simulink model "matlab model"  (R2023a)
settings: Solver=ode4  StartTime=0.0  StopTime=0.15  FixedStep=1e-6  RelTol=1e-3  EnableMultiTasking=on
libraries: neural x15, spsMosfetLib x15, simulink x10, spsMeanLib x6, spsSeriesRLCBranchLib x4, spsVoltageMeasurementLib x3, spsDCVoltageSourceLib x2, spsThreePhaseVIMeasurementLib x1, sps_lib x1
(part 1 of 2)
settings Model: Creator=VENUS  LastModifiedBy=air
settings SolverCC: AlgebraicLoopSolver=TrustRegion
settings DataIOCC: LimitDataPoints=on  SaveFormat=Array  ReturnWorkspaceOutputs=off
settings OptimizationCC: LifeSpan=inf
settings DebuggingCC: SolverPrmCheckMsg=warning  UnconnectedInputMsg=warning  UnconnectedOutputMsg=warning  UnconnectedLineMsg=warning  SFUnexpectedBacktrackingDiag=warning  SFNoUnconditionalDefaultTransitionDiag=warning  SFExecutionAtInitializationDiag=none  ArithmeticOperatorsInVariantConditions=warning
settings HardwareCC: ProdBitPerPointer=32  ProdBitPerSizeT=32  ProdBitPerPtrDiffT=32  ProdLargestAtomicFloat=None  ProdIntDivRoundTo=Undefined  ProdEndianess=Unspecified  ProdWordSize=32  ProdHWDeviceType=32-bit Generic
settings ModelReferenceCC: EnableRefExpFcnMdlSchedulingChecks=on  PropagateSignalLabelsOutOfModel=off
settings SFSimCC: SimUseLocalCustomCode=off  CustomCodeUndefinedFunction=UseInterfaceOnly
settings RTWCC: RTWUseLocalCustomCode=off
settings CodeAppCC: StateflowObjectComments=on
settings GRTTargetCC: TargetLangStandard=C89/C90 (ANSI)
settings ConfigComp: CovMetricSettings=dw  CovSaveCumulativeToWorkspaceVar=on  CovSaveSingleToWorkspaceVar=on  CovExternalEMLEnable=off  CovSFcnEnable=off
settings SimscapeCC: SimscapeNormalizeSystem=off

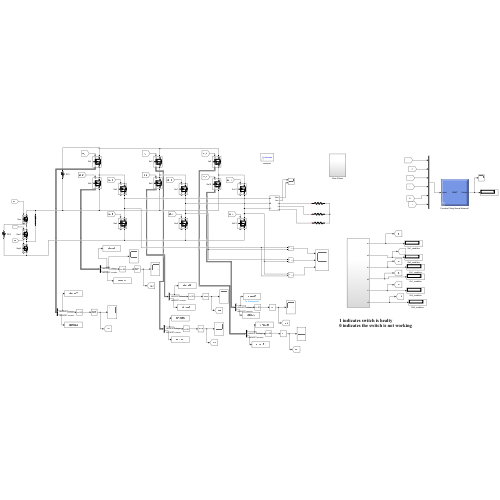
[thumbnail: Simulink's stored preview of the top-level diagram]
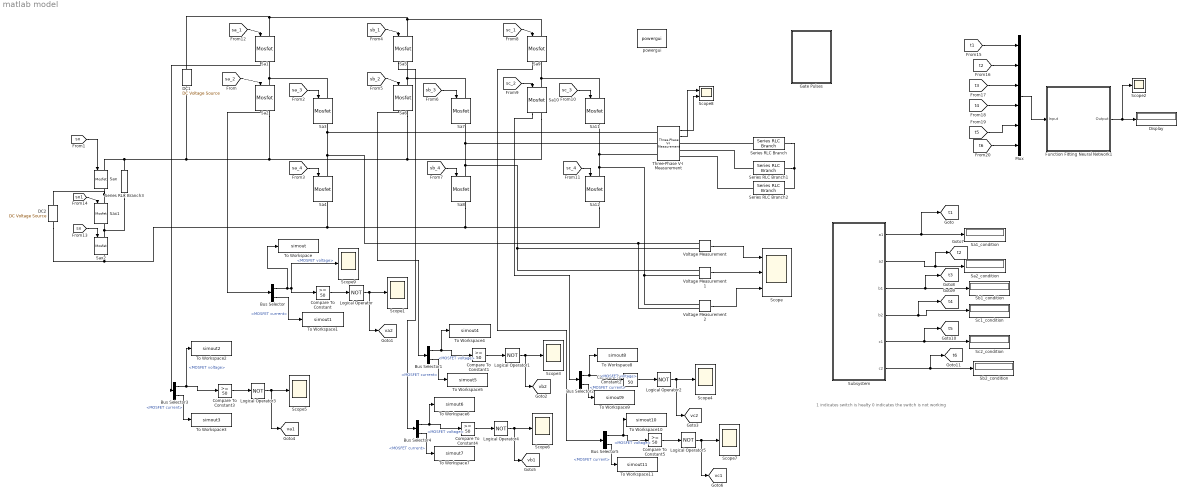
== system matlab model ==
  note: 1 indicates switch is healty
      | 0 indicates the switch is not working
  Bus Selector{,1..5} (6 alike) : BusSelector  OutputSignals=MOSFET voltage,MOSFET current
  Compare To Constant{,1..5} (6 alike) : simulink/Logic and Bit Operations/Compare To Constant  relop=>=  const=50  OutDataTypeStr=boolean
  DC1 : spsDCVoltageSourceLib/DC Voltage Source  Amplitude=300  Measurements=None
  DC2 : spsDCVoltageSourceLib/DC Voltage Source  Amplitude=300  Measurements=None
  Display : Display
  Function Fitting Neural Network1 : Subsystem
      mask help: Function Fitting Neural Network
      mask Display: e = 0.06;c1 = [120 150 230]/255;c2 = ([120 150 230]+0)/383;c3 = ([120 150 230]+128)/383;patch([0 1 1 0],[0 0 1 1],c1);patch([0 1 1 1-e 1-e 0+e],[0 0 1 1-e 0+e 0+e],c2);patch([0 0 1 1-e 0+e 0+e],[0 1 1 1-e 1-e 0+e],c3);plot([0 1 1 0 0],[0 0 1 1 0]);fprintf('NNET');port_label('input',1,' Input');port_label('output',1,'Output ');
  Gate Pulses : Subsystem
  Logical Operator{,1..5} (6 alike) : Logic  Operator=NOT  AllPortsSameDT=off  OutDataTypeStr=boolean
  Mux : Mux  Inputs=6
  Sa{1..12} (12 alike) : spsMosfetLib/Mosfet  Ron=0.1  Lon=0  Rd=0.01  Vfd=0  IC=0  Rs=1e5  Cs=inf  Measurements=on
  Sa1_condition : Display
  Sa2_condition : Display
  Sax : spsMosfetLib/Mosfet  Ron=0.1  Lon=0  Rd=0.01  Vfd=0  IC=0  Rs=1e5  Cs=inf  Measurements=on
  Sax1 : spsMosfetLib/Mosfet  Ron=0.1  Lon=0  Rd=0.01  Vfd=0  IC=0  Rs=1e5  Cs=inf  Measurements=on
  Sax2 : spsMosfetLib/Mosfet  Ron=0.1  Lon=0  Rd=0.01  Vfd=0  IC=0  Rs=1e5  Cs=inf  Measurements=on
  Sb1_condition : Display
  Sb2_condition : Display
  Sc1_condition : Display
  Sc2_condition : Display
  Scope : Scope  NumInputPorts=3
  Scope{1..7,9} (8 alike) : Scope
  Scope8 : Scope  NumInputPorts=2
  Series RLC Branch : spsSeriesRLCBranchLib/Series RLC Branch  LConnTagsString=__new0  RConnTagsString=__new0  BranchType=R  Resistance=100  Inductance=1e-3  SetiL0=off  InitialCurrent=0  Capacitance=1e-6  Setx0=off  InitialVoltage=0  Measurements=None
  Series RLC Branch1 : spsSeriesRLCBranchLib/Series RLC Branch  LConnTagsString=__new0  RConnTagsString=__new0  BranchType=R  Resistance=100  Inductance=1e-3  SetiL0=off  InitialCurrent=0  Capacitance=1e-6  Setx0=off  InitialVoltage=0  Measurements=None
  Series RLC Branch2 : spsSeriesRLCBranchLib/Series RLC Branch  LConnTagsString=__new0  RConnTagsString=__new0  BranchType=R  Resistance=100  Inductance=1e-3  SetiL0=off  InitialCurrent=0  Capacitance=1e-6  Setx0=off  InitialVoltage=0  Measurements=None
  Series RLC Branch3 : spsSeriesRLCBranchLib/Series RLC Branch  LConnTagsString=__new0  RConnTagsString=__new0  BranchType=RC  Resistance=0.01  Inductance=1e-3  SetiL0=off  InitialCurrent=0  Capacitance=1000e-6  Setx0=off  InitialVoltage=0  Measurements=None
  Subsystem : Subsystem
  Three-Phase V-I Measurement : spsThreePhaseVIMeasurementLib/Three-Phase V-I Measurement  VoltageMeasurement=phase-to-phase  SetLabelV=off  LabelV=Vabc  Vpu=off  VpuLL=off  CurrentMeasurement=yes  SetLabelI=off  LabelI=Iabc  Ipu=off  Pbase=100e6  Vbase=500e3  OutputType=Complex  PhasorSimulation=off  PSBequivalent=0
  To Workspace : ToWorkspace  VariableName=simout  SaveFormat=Timeseries  SampleTime=-1
  To Workspace1 : ToWorkspace  VariableName=simout1  SaveFormat=Timeseries  SampleTime=-1
  To Workspace10 : ToWorkspace  VariableName=simout10  SaveFormat=Timeseries  SampleTime=-1
  To Workspace11 : ToWorkspace  VariableName=simout11  SaveFormat=Timeseries  SampleTime=-1
  To Workspace2 : ToWorkspace  VariableName=simout2  SaveFormat=Timeseries  SampleTime=-1
  To Workspace3 : ToWorkspace  VariableName=simout3  SaveFormat=Timeseries  SampleTime=-1
  To Workspace4 : ToWorkspace  VariableName=simout4  SaveFormat=Timeseries  SampleTime=-1
  To Workspace5 : ToWorkspace  VariableName=simout5  SaveFormat=Timeseries  SampleTime=-1
  To Workspace6 : ToWorkspace  VariableName=simout6  SaveFormat=Timeseries  SampleTime=-1
  To Workspace7 : ToWorkspace  VariableName=simout7  SaveFormat=Timeseries  SampleTime=-1
  To Workspace8 : ToWorkspace  VariableName=simout8  SaveFormat=Timeseries  SampleTime=-1
  To Workspace9 : ToWorkspace  VariableName=simout9  SaveFormat=Timeseries  SampleTime=-1
  Voltage Measurement : spsVoltageMeasurementLib/Voltage Measurement  PhasorSimulation=off  OutputType=Complex  PSBequivalent=0
  Voltage Measurement1 : spsVoltageMeasurementLib/Voltage Measurement  PhasorSimulation=off  OutputType=Complex  PSBequivalent=0
  Voltage Measurement2 : spsVoltageMeasurementLib/Voltage Measurement  PhasorSimulation=off  OutputType=Complex  PSBequivalent=0
  powergui : sps_lib/powergui  Priority=1  SimulationMode=Continuous  SampleTime=50e-6  frequency=60  Iterations=50  frequencyindice=0  Pbase=100e6  ErrMax=1e-4  UnitsV=kV  UnitsW=MW  buscounter=0  FunctionMessages=off  echomessages=off  EnableUseOfTLC=off  CurrentSourceSwitches=on  DisableSnubberDevices=off  DisableRonSwitches=off  DisableVfSwitches=off  DisplayEquations=off  AutomaticDiscreteSolvers=off  SolverType=Tustin  Interpol=off  ExternalGateDelay=off  methode=off  Ts=0  x0status=blocks  SPID=off  SwTol=0  HookPort=off  NonlinearTolerance=1e-4  nMaxIteration=100  ContinueOnMaxIteration=off  RestoreLinks=warning  ResistiveCurrentMeasurement=off  Frange=[0:2:500]  Ylog=off  Xlog=on  ShowGrid=off  save=off  variable=ZData  structure=0  ZoomFFT=off  StartTime=0.0  cycles=1  DisplayStyle=1  fundamental=60  FreqAxis=off  MaxFrequency=1000  frequencyindicesteady=1  RmsSteady=1  display=off
  tag scope: t1=global, t2=global, t3=global, t4=global, t5=global, t6=global, va1=global, va2=global, vb1=global, vb2=global, vc1=global, vc2=global
  wires:
  [sa_3] -> Sa3/1
  [sa_4] -> Sa4/1
  [sb_4] -> Sa8/1
  [sb_3] -> Sa7/1
  [sb_2] -> Sa6/1
  [sb_1] -> Sa5/1
  [sc_1] -> Sa9/1
  [sc_2] -> Sa10/1
  [sc_4] -> Sa12/1
  [sc_3] -> Sa11/1
  Voltage Measurement1/1 -> Scope/2
  Voltage Measurement/1 -> Scope/1
  Voltage Measurement2/1 -> Scope/3
  Sa2/1 -> Bus Selector/1
  Bus Selector/1 -> To Workspace/1, Compare To Constant/1, Scope9/1  "<MOSFET voltage>"
  Compare To Constant/1 -> Logical Operator/1
  Logical Operator/1 -> [va2], Scope1/1
  Sa6/1 -> Bus Selector1/1
  Bus Selector1/1 -> To Workspace4/1, Compare To Constant1/1  "<MOSFET voltage>"
  Compare To Constant1/1 -> Logical Operator1/1
  Logical Operator1/1 -> [vb2], Scope3/1
  Sa10/1 -> Bus Selector2/1
  Bus Selector2/1 -> To Workspace8/1, Compare To Constant2/1  "<MOSFET voltage>"
  Compare To Constant2/1 -> Logical Operator2/1
  Logical Operator2/1 -> [vc2], Scope4/1
  Sa1/1 -> Bus Selector3/1
  Bus Selector3/1 -> To Workspace2/1, Compare To Constant3/1  "<MOSFET voltage>"
  Compare To Constant3/1 -> Logical Operator3/1
  Logical Operator3/1 -> Scope5/1, [va1]
  Sa5/1 -> Bus Selector4/1
  Bus Selector4/1 -> To Workspace6/1, Compare To Constant4/1  "<MOSFET voltage>"
  Compare To Constant4/1 -> Logical Operator4/1
  Logical Operator4/1 -> Scope6/1, [vb1]
  Bus Selector5/1 -> To Workspace10/1, Compare To Constant5/1  "<MOSFET voltage>"
  Compare To Constant5/1 -> Logical Operator5/1
  Logical Operator5/1 -> Scope7/1, [vc1]
  [sa_2] -> Sa2/1
  [sa_1] -> Sa1/1
  Sa9/1 -> Bus Selector5/1
  Three-Phase V-I Measurement/2 -> Scope8/1
  Three-Phase V-I Measurement/1 -> Scope8/2
  Subsystem/1(a1) -> [t1], Sa1_condition/1
  Subsystem/2(a2) -> [t2], Sa2_condition/1
  Subsystem/4(b2) -> [t4], Sc1_condition/1
  Subsystem/6(c2) -> [t6], Sb2_condition/1
  [sx] -> Sax/1
  [sx] -> Sax2/1
  [sx1] -> Sax1/1
  Subsystem/3(b1) -> [t3], Sb1_condition/1
  Subsystem/5(c1) -> [t5], Sc2_condition/1
  [t1] -> Mux/1
  [t2] -> Mux/2
  [t3] -> Mux/3
  [t4] -> Mux/4
  [t5] -> Mux/5
  [t6] -> Mux/6
  Mux/1 -> Function Fitting Neural Network1/1(Input)
  Function Fitting Neural Network1/1(Output) -> Scope2/1, Display/1
  Bus Selector/2 -> To Workspace1/1  "<MOSFET current>"
  Bus Selector3/2 -> To Workspace3/1  "<MOSFET current>"
  Bus Selector1/2 -> To Workspace5/1  "<MOSFET current>"
  Bus Selector4/2 -> To Workspace7/1  "<MOSFET current>"
  Bus Selector2/2 -> To Workspace9/1  "<MOSFET current>"
  Bus Selector5/2 -> To Workspace11/1  "<MOSFET current>"
  connections:
  Sa2/LConn1 -- Sa3/LConn1 -- Sa1/RConn1
  DC1/RConn1 -- Sa9/LConn1 -- Sa5/LConn1 -- Sa1/LConn1
  Sa4/LConn1 -- Voltage Measurement2/LConn2 -- Voltage Measurement/LConn1 -- Three-Phase V-I Measurement/LConn1 -- Sa3/RConn1
  Sa7/LConn1 -- Sa6/LConn1 -- Sa5/RConn1
  Sa8/LConn1 -- Voltage Measurement1/LConn1 -- Voltage Measurement/LConn2 -- Three-Phase V-I Measurement/LConn2 -- Sa7/RConn1
  Sa10/LConn1 -- Sa11/LConn1 -- Sa9/RConn1
  Sa12/LConn1 -- Three-Phase V-I Measurement/LConn3 -- Sa11/RConn1 -- Voltage Measurement2/LConn1 -- Voltage Measurement1/LConn2
  Series RLC Branch/LConn1 -- Three-Phase V-I Measurement/RConn1
  Series RLC Branch2/LConn1 -- Three-Phase V-I Measurement/RConn3
  Series RLC Branch1/LConn1 -- Three-Phase V-I Measurement/RConn2
  Series RLC Branch/RConn1 -- Series RLC Branch1/RConn1 -- Series RLC Branch2/RConn1
  Sax1/LConn1 -- DC2/RConn1 -- Sax/RConn1
  Sax2/LConn1 -- Series RLC Branch3/RConn1 -- Sax1/RConn1
  Sa2/RConn1 -- Sa10/RConn1 -- Sa6/RConn1 -- Sax/LConn1 -- Series RLC Branch3/LConn1 -- DC1/LConn1
  Sa12/RConn1 -- Sa8/RConn1 -- DC2/LConn1 -- Sax2/RConn1 -- Sa4/RConn1

== system matlab model/Function Fitting Neural Network1 ==
  Input : Inport  PortDimensions=6
      mask Display: e = 0.06;c1 = [120 230 180]/255;c2 = ([120 230 180]+0)/(256+128);c3 = ([120 230 180]+128)/(256+128);patch([0 1 1 0],[0 0 1 1],c1);patch([0 1 1 1-e 1-e 0+e],[0 0 1 1-e 0+e 0+e],c2);patch([0 0 1 1-e 0+e 0+e],[0 1 1 1-e 1-e 0+e],c3);plot([0 1 1 0 0],[0 0 1 1 0]);
  Layer 1 : Subsystem
      mask Display: e = 0.06;c1 = [120 150 230]/255;c2 = ([120 150 230]+0)/383;c3 = ([120 150 230]+128)/383;patch([0 1 1 0],[0 0 1 1],c1);patch([0 1 1 1-e 1-e 0+e],[0 0 1 1-e 0+e 0+e],c2);patch([0 0 1 1-e 0+e 0+e],[0 1 1 1-e 1-e 0+e],c3);plot([0 1 1 0 0],[0 0 1 1 0]);
  Layer 2 : Subsystem
      mask Display: e = 0.06;c1 = [120 150 230]/255;c2 = ([120 150 230]+0)/383;c3 = ([120 150 230]+128)/383;patch([0 1 1 0],[0 0 1 1],c1);patch([0 1 1 1-e 1-e 0+e],[0 0 1 1-e 0+e 0+e],c2);patch([0 0 1 1-e 0+e 0+e],[0 1 1 1-e 1-e 0+e],c3);plot([0 1 1 0 0],[0 0 1 1 0]);
  Process Input 1 : Subsystem
      mask Display: e = 0.06;c1 = [120 150 230]/255;c2 = ([120 150 230]+0)/383;c3 = ([120 150 230]+128)/383;patch([0 1 1 0],[0 0 1 1],c1);patch([0 1 1 1-e 1-e 0+e],[0 0 1 1-e 0+e 0+e],c2);patch([0 0 1 1-e 0+e 0+e],[0 1 1 1-e 1-e 0+e],c3);plot([0 1 1 0 0],[0 0 1 1 0]);
  Process Output 1 : Subsystem
      mask Display: e = 0.06;c1 = [120 150 230]/255;c2 = ([120 150 230]+0)/383;c3 = ([120 150 230]+128)/383;patch([0 1 1 0],[0 0 1 1],c1);patch([0 1 1 1-e 1-e 0+e],[0 0 1 1-e 0+e 0+e],c2);patch([0 0 1 1-e 0+e 0+e],[0 1 1 1-e 1-e 0+e],c3);plot([0 1 1 0 0],[0 0 1 1 0]);
  Output : Outport  InitialOutput=0
      mask Display: e = 0.06;c1 = [120 230 180]/255;c2 = ([120 230 180]+0)/(256+128);c3 = ([120 230 180]+128)/(256+128);patch([0 1 1 0],[0 0 1 1],c1);patch([0 1 1 1-e 1-e 0+e],[0 0 1 1-e 0+e 0+e],c2);patch([0 0 1 1-e 0+e 0+e],[0 1 1 1-e 1-e 0+e],c3);plot([0 1 1 0 0],[0 0 1 1 0]);
  wires:
  Input/1 -> Process Input 1/1(x)
  Process Output 1/1(y) -> Output/1
  Process Input 1/1(p) -> Layer 1/1("p{1}")
  Layer 1/1("a{1}") -> [feedback1]
  [feedback1] -> Layer 2/1("a{1} ")
  Layer 2/1("a{2}") -> Process Output 1/1(a)

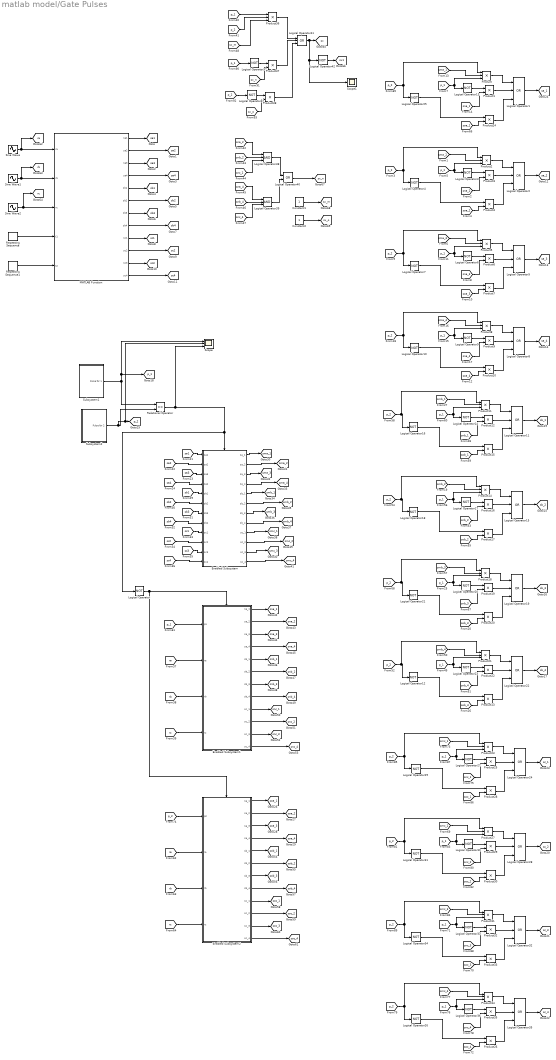
== system matlab model/Gate Pulses ==
  Constant1 : Constant
  Constant2 : Constant
  Enabled Subsystem : Subsystem  TreatAsAtomicUnit=on
  Enabled Subsystem1 : Subsystem  TreatAsAtomicUnit=on
  Enabled Subsystem2 : Subsystem  TreatAsAtomicUnit=on
  Logical Operator{,3..4,6..7,9..10,12..14,16..18,20..21,23,25..27,29..31,33..34,36..37,42..43} (28 alike) : Logic  Operator=NOT  AllPortsSameDT=off  OutDataTypeStr=boolean
  Logical Operator{1..2,5,8,11,15,19,22,24,28,32,35,41} (13 alike) : Logic  Operator=OR  Inputs=3  AllPortsSameDT=off  OutDataTypeStr=boolean
  Logical Operator38 : Logic  Inputs=3  AllPortsSameDT=off  OutDataTypeStr=boolean
  Logical Operator39 : Logic  Inputs=3  AllPortsSameDT=off  OutDataTypeStr=boolean
  Logical Operator40 : Logic  Operator=OR  AllPortsSameDT=off  OutDataTypeStr=boolean
  MATLAB Function : MATLAB Function  TreatAsAtomicUnit=on
  Product{,2,5,8,11,14,18,21,23,27,31,34,36} (13 alike) : Product  Inputs=3
  Product{1,3..4,6..7,9..10,12..13,15..17,19..20,22,24..26,28..30,32..33,35,37..38} (26 alike) : Product
  Relational Operator : RelationalOperator  Operator===  OutDataTypeStr=boolean  InputSameDT=off
  Repeating Sequence : simulink/Sources/Repeating Sequence  rep_seq_t=[0 1/2000 1/1000]  rep_seq_y=[0 1 0]
  Repeating Sequence1 : simulink/Sources/Repeating Sequence  rep_seq_t=[0 1/2000 1/1000]  rep_seq_y=[-1 0 -1]
  Scope : Scope  NumInputPorts=3
  Scope1 : Scope
  Sine Wave : Sin  Amplitude=.8  Frequency=100*pi  SampleTime=0
  Sine Wave1 : Sin  Amplitude=.8  Frequency=100*pi  Phase=2*pi/3  SampleTime=0
  Sine Wave2 : Sin  Amplitude=.8  Frequency=100*pi  Phase=4*pi/3  SampleTime=0
  Subsystem1 : Subsystem
  Subsystem2 : Subsystem
  tag scope: p_1=global, p_2=global, ra=global, rb=global, rc=global, sa1=global, sa2=global, sa3=global, sa4=global, sa_1=global, sa_2=global, sa_3=global, sa_4=global, sb1=global, sb2=global, sb3=global, sb4=global, sb_1=global, sb_2=global, sb_3=global, sb_4=global, sc1=global, sc2=global, sc3=global, sc4=global, sc_1=global, sc_2=global, sc_3=global, sc_4=global, sma_1=global, sma_2=global, sma_3=global, sma_4=global, smb_1=global, smb_2=global, smb_3=global, smb_4=global, smc_1=global, smc_2=global, smc_3=global, smc_4=global, sna_1=global, sna_2=global, sna_3=global, sna_4=global, snb_1=global, snb_2=global, snb_3=global, snb_4=global, snc_1=global, snc_2=global, snc_3=global, snc_4=global, soa_1=global, soa_2=global, soa_3=global, soa_4=global, sob_1=global, sob_2=global, sob_3=global, sob_4=global, soc_1=global, soc_2=global, soc_3=global, soc_4=global, sx1=global, sx=global, sx_m=global, sx_n=global, sx_o=global
  wires:
  Sine Wave/1 -> [ra], MATLAB Function/1(ra)
  Sine Wave1/1 -> [rb], MATLAB Function/2(rb)
  Repeating Sequence/1 -> MATLAB Function/4(t1)
  MATLAB Function/2(sa2) -> [sa2]
  MATLAB Function/9(sc1) -> [sc1]
  MATLAB Function/4(sa4) -> [sa4]
  MATLAB Function/10(sc2) -> [sc2]
  MATLAB Function/12(sc4) -> [sc4]
  MATLAB Function/5(sb1) -> [sb1]
  MATLAB Function/6(sb2) -> [sb2]
  MATLAB Function/7(sb3) -> [sb3]
  MATLAB Function/8(sb4) -> [sb4]
  Sine Wave2/1 -> [rc], MATLAB Function/3(rc)
  MATLAB Function/3(sa3) -> [sa3]
  MATLAB Function/11(sc3) -> [sc3]
  MATLAB Function/1(sa1) -> [sa1]
  Repeating Sequence1/1 -> MATLAB Function/5(t2)
  Product/1 -> Logical Operator1/1
  Product1/1 -> Logical Operator1/2
  Logical Operator1/1 -> [sa_1]
  Subsystem1/1(Pulse for 1) -> Relational Operator/1, Scope/1, [p_1]
  Subsystem2/1(Pulse for 2) -> Scope/2, [p_2], Relational Operator/2
  Relational Operator/1 -> Scope/3, Logical Operator/1, Enabled Subsystem/Enable
  [sa1] -> Enabled Subsystem/1(sa1)
  [sa2] -> Enabled Subsystem/2(sa2)
  [sa3] -> Enabled Subsystem/3(sa3)
  [sa4] -> Enabled Subsystem/4(sa4)
  [sb2] -> Enabled Subsystem/6(sb2)
  [sb4] -> Enabled Subsystem/8(sb4)
  [sb1] -> Enabled Subsystem/5(sb1)
  [sb3] -> Enabled Subsystem/7(sb3)
  [sc2] -> Enabled Subsystem/10(sc2)
  [sc4] -> Enabled Subsystem/12(sc4)
  [sc3] -> Enabled Subsystem/11(sc3)
  [sc1] -> Enabled Subsystem/9(sc1)
  Enabled Subsystem/1(sa_1) -> [sma_1]
  Enabled Subsystem/2(sa_2) -> [sma_2]
  Enabled Subsystem/3(sa_3) -> [sma_3]
  Enabled Subsystem/4(sa_4) -> [sma_4]
  Enabled Subsystem/5(sb_1) -> [smb_1]
  Enabled Subsystem/6(sb_2) -> [smb_2]
  Enabled Subsystem/7(sb_3) -> [smb_3]
  Enabled Subsystem/8(sb_4) -> [smb_4]
  Enabled Subsystem/10(sc_2) -> [smc_2]
  Enabled Subsystem/11(sc_3) -> [smc_3]
  Enabled Subsystem/12(sc_4) -> [smc_4]
  Enabled Subsystem/9(sc_1) -> [smc_1]
  Enabled Subsystem1/2(sa_2) -> [sna_2]
  Enabled Subsystem1/4(sa_4) -> [sna_4]
  Enabled Subsystem1/5(sb_1) -> [snb_1]
  Enabled Subsystem1/6(sb_2) -> [snb_2]
  Enabled Subsystem1/7(sb_3) -> [snb_3]
  Enabled Subsystem1/8(sb_4) -> [snb_4]
  Enabled Subsystem1/10(sc_2) -> [snc_2]
  Enabled Subsystem1/11(sc_3) -> [snc_3]
  Enabled Subsystem1/12(sc_4) -> [snc_4]
  Enabled Subsystem1/9(sc_1) -> [snc_1]
  Enabled Subsystem1/1(sa_1) -> [sna_1]
  Enabled Subsystem1/3(sa_3) -> [sna_3]
  [sna_1] -> Product1/2
  Logical Operator13/1 -> Product1/1
  [p_1] -> Logical Operator13/1, Product/3
  [p_1] -> Enabled Subsystem1/1(p1)
  Logical Operator/1 -> Enabled Subsystem1/Enable, Enabled Subsystem2/Enable
  Enabled Subsystem2/2(sa_2) -> [soa_2]
  Enabled Subsystem2/4(sa_4) -> [soa_4]
  Enabled Subsystem2/5(sb_1) -> [sob_1]
  Enabled Subsystem2/6(sb_2) -> [sob_2]
  Enabled Subsystem2/7(sb_3) -> [sob_3]
  Enabled Subsystem2/8(sb_4) -> [sob_4]
  Enabled Subsystem2/10(sc_2) -> [soc_2]
  Enabled Subsystem2/11(sc_3) -> [soc_3]
  Enabled Subsystem2/12(sc_4) -> [soc_4]
  Enabled Subsystem2/9(sc_1) -> [soc_1]
  Enabled Subsystem2/1(sa_1) -> [soa_1]
  Enabled Subsystem2/3(sa_3) -> [soa_3]
  [p_2] -> Enabled Subsystem2/1(p2)
  [ra] -> Enabled Subsystem2/2(ra)
  [rb] -> Enabled Subsystem2/3(rb)
  [rc] -> Enabled Subsystem2/4(rc)
  [p_2] -> Product/1, Logical Operator25/1
  [sma_1] -> Product/2
  Logical Operator25/1 -> Product24/1
  [soa_1] -> Product24/2
  Product24/1 -> Logical Operator1/3
  Product2/1 -> Logical Operator2/1
  Product3/1 -> Logical Operator2/2
  Logical Operator2/1 -> [sa_2]
  [sna_2] -> Product3/2
  Logical Operator3/1 -> Product3/1
  [p_1] -> Product2/3, Logical Operator3/1
  [p_2] -> Logical Operator4/1, Product2/1
  [sma_2] -> Product2/2
  Logical Operator4/1 -> Product4/1
  [soa_2] -> Product4/2
  Product4/1 -> Logical Operator2/3
  Product5/1 -> Logical Operator5/1
  Product6/1 -> Logical Operator5/2
  Logical Operator5/1 -> [sa_3]
  [sna_3] -> Product6/2
  Logical Operator6/1 -> Product6/1
  [p_1] -> Logical Operator6/1, Product5/3
  [p_2] -> Product5/1, Logical Operator7/1
  [sma_3] -> Product5/2
  Logical Operator7/1 -> Product7/1
  [soa_3] -> Product7/2
  Product7/1 -> Logical Operator5/3
  Product8/1 -> Logical Operator8/1
  Product9/1 -> Logical Operator8/2
  Logical Operator8/1 -> [sa_4]
  [sna_4] -> Product9/2
  Logical Operator9/1 -> Product9/1
  [p_1] -> Product8/3, Logical Operator9/1
  [p_2] -> Logical Operator10/1, Product8/1
  [sma_4] -> Product8/2
  Logical Operator10/1 -> Product10/1
  [soa_4] -> Product10/2
  Product10/1 -> Logical Operator8/3
  Product11/1 -> Logical Operator11/1
  Product12/1 -> Logical Operator11/2
  Logical Operator11/1 -> [sb_1]
  [snb_1] -> Product12/2
  Logical Operator14/1 -> Product12/1
  [p_1] -> Product11/3, Logical Operator14/1
  [p_2] -> Logical Operator16/1, Product11/1
  [smb_1] -> Product11/2
  Logical Operator16/1 -> Product15/1
  [sob_1] -> Product15/2
  Product15/1 -> Logical Operator11/3
  Product14/1 -> Logical Operator15/1
  Product16/1 -> Logical Operator15/2
  Logical Operator15/1 -> [sb_2]
  [snb_2] -> Product16/2
  Logical Operator17/1 -> Product16/1
  [p_1] -> Logical Operator17/1, Product14/3
  [p_2] -> Product14/1, Logical Operator18/1
  [smb_2] -> Product14/2
  Logical Operator18/1 -> Product17/1
  [sob_2] -> Product17/2
  Product17/1 -> Logical Operator15/3
  Product18/1 -> Logical Operator19/1
  Product19/1 -> Logical Operator19/2
  Logical Operator19/1 -> [sb_3]
  [snb_3] -> Product19/2
  Logical Operator20/1 -> Product19/1
  [p_1] -> Product18/3, Logical Operator20/1
  [p_2] -> Logical Operator21/1, Product18/1
  [smb_3] -> Product18/2
  Logical Operator21/1 -> Product20/1
  [sob_3] -> Product20/2
  Product20/1 -> Logical Operator19/3
  Product21/1 -> Logical Operator22/1
  Product22/1 -> Logical Operator22/2
  Logical Operator22/1 -> [sb_4]
  [snb_4] -> Product22/2
  Logical Operator23/1 -> Product22/1
  [p_1] -> Logical Operator23/1, Product21/3
  [p_2] -> Product21/1, Logical Operator12/1
  [smb_4] -> Product21/2
  Logical Operator12/1 -> Product13/1
  [sob_4] -> Product13/2
  Product13/1 -> Logical Operator22/3
  Product23/1 -> Logical Operator24/1
  Product25/1 -> Logical Operator24/2
  Logical Operator24/1 -> [sc_1]
  [snc_1] -> Product25/2
  Logical Operator27/1 -> Product25/1
  [p_1] -> Logical Operator27/1, Product23/3
  [p_2] -> Product23/1, Logical Operator29/1
  [smc_1] -> Product23/2
  Logical Operator29/1 -> Product28/1
  [soc_1] -> Product28/2
  Product28/1 -> Logical Operator24/3
  Product27/1 -> Logical Operator28/1
  Product29/1 -> Logical Operator28/2
  Logical Operator28/1 -> [sc_2]
  [snc_2] -> Product29/2
  Logical Operator30/1 -> Product29/1
  [p_1] -> Product27/3, Logical Operator30/1
  [p_2] -> Logical Operator31/1, Product27/1
  [smc_2] -> Product27/2
  Logical Operator31/1 -> Product30/1
  [soc_2] -> Product30/2
  Product30/1 -> Logical Operator28/3
  Product31/1 -> Logical Operator32/1
  Product32/1 -> Logical Operator32/2
  Logical Operator32/1 -> [sc_3]
  [snc_3] -> Product32/2
  Logical Operator33/1 -> Product32/1
  [p_1] -> Logical Operator33/1, Product31/3
  [p_2] -> Product31/1, Logical Operator34/1
  [smc_3] -> Product31/2
  Logical Operator34/1 -> Product33/1
  [soc_3] -> Product33/2
  Product33/1 -> Logical Operator32/3
  Product34/1 -> Logical Operator35/1
  Product35/1 -> Logical Operator35/2
  Logical Operator35/1 -> [sc_4]
  [snc_4] -> Product35/2
  Logical Operator36/1 -> Product35/1
  [p_1] -> Product34/3, Logical Operator36/1
  [p_2] -> Logical Operator26/1, Product34/1
  [smc_4] -> Product34/2
  Logical Operator26/1 -> Product26/1
  [soc_4] -> Product26/2
  Product26/1 -> Logical Operator35/3
  [ra] -> Enabled Subsystem1/2(ra)
  [rb] -> Enabled Subsystem1/3(rb)
  [rc] -> Enabled Subsystem1/4(rc)
  [p_1] -> Product36/1
  [p_2] -> Product36/2
  [sx_m] -> Product36/3
  [snb_2] -> Logical Operator38/2
  [sna_2] -> Logical Operator38/1
  [snc_2] -> Logical Operator38/3
  [snc_4] -> Logical Operator39/3
  [sna_4] -> Logical Operator39/1
  [snb_4] -> Logical Operator39/2
  Logical Operator38/1 -> Logical Operator40/1
  Logical Operator39/1 -> Logical Operator40/2
  Logical Operator40/1 -> [sx_n]
  Constant1/1 -> [sx_m]
  [p_1] -> Logical Operator37/1
  Logical Operator37/1 -> Product37/1
  [sx_n] -> Product37/2
  Product36/1 -> Logical Operator41/1
  Product37/1 -> Logical Operator41/2
  Logical Operator41/1 -> Scope1/1, Logical Operator42/1, [sx]
  Logical Operator42/1 -> [sx1]
  Constant2/1 -> [sx_o]
  Product38/1 -> Logical Operator41/3
  [sx_o] -> Product38/2
  Logical Operator43/1 -> Product38/1
  [p_2] -> Logical Operator43/1

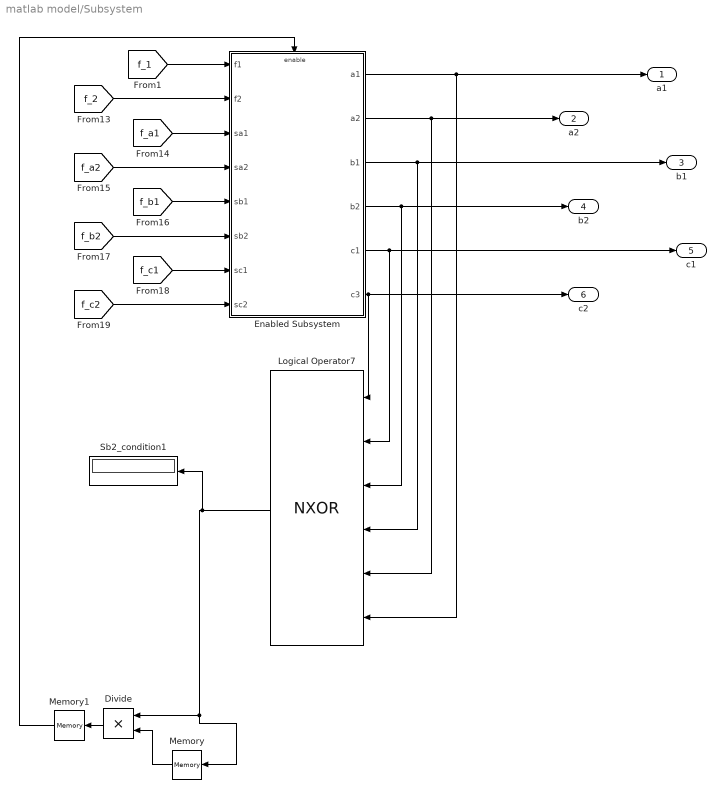
== system matlab model/Subsystem ==
  Divide : Product  Inputs=**
  Enabled Subsystem : Subsystem  TreatAsAtomicUnit=on
  Logical Operator7 : Logic  Operator=NXOR  Inputs=6  AllPortsSameDT=off  OutDataTypeStr=boolean
  Memory : Memory  InitialCondition=1
  Memory1 : Memory  InitialCondition=1
  Sb2_condition1 : Display
  a1 : Outport  VectorParamsAs1DForOutWhenUnconnected=off
  a2 : Outport  Port=2  VectorParamsAs1DForOutWhenUnconnected=off
  b1 : Outport  Port=3  VectorParamsAs1DForOutWhenUnconnected=off
  b2 : Outport  Port=4  VectorParamsAs1DForOutWhenUnconnected=off
  c1 : Outport  Port=5  VectorParamsAs1DForOutWhenUnconnected=off
  c2 : Outport  Port=6  VectorParamsAs1DForOutWhenUnconnected=off
  wires:
  Memory/1 -> Divide/2
  Logical Operator7/1 -> Sb2_condition1/1, Memory/1, Divide/1
  Enabled Subsystem/3(b1) -> b1/1, Logical Operator7/4
  Enabled Subsystem/4(b2) -> b2/1, Logical Operator7/3
  Enabled Subsystem/2(a2) -> a2/1, Logical Operator7/5
  Divide/1 -> Memory1/1
  Enabled Subsystem/6(c3) -> c2/1, Logical Operator7/1
  Enabled Subsystem/5(c1) -> c1/1, Logical Operator7/2
  Enabled Subsystem/1(a1) -> a1/1, Logical Operator7/6
  [f_a2] -> Enabled Subsystem/4(sa2)
  [f_b2] -> Enabled Subsystem/6(sb2)
  [f_b1] -> Enabled Subsystem/5(sb1)
  [f_c1] -> Enabled Subsystem/7(sc1)
  [f_c2] -> Enabled Subsystem/8(sc2)
  [f_a1] -> Enabled Subsystem/3(sa1)
  [f_1] -> Enabled Subsystem/1(f1)
  [f_2] -> Enabled Subsystem/2(f2)
  Memory1/1 -> Enabled Subsystem/Enable

== system matlab model/Function Fitting Neural Network1/Layer 1 ==
  "p{1}" : Inport  PortDimensions=6
      mask Display: e = 0.06;c1 = [120 230 180]/255;c2 = ([120 230 180]+0)/(256+128);c3 = ([120 230 180]+128)/(256+128);patch([0 1 1 0],[0 0 1 1],c1);patch([0 1 1 1-e 1-e 0+e],[0 0 1 1-e 0+e 0+e],c2);patch([0 0 1 1-e 0+e 0+e],[0 1 1 1-e 1-e 0+e],c3);plot([0 1 1 0 0],[0 0 1 1 0]);
  Delays 1 : Subsystem
      mask Display: e = 0.06;c1 = [120 150 230]/255;c2 = ([120 150 230]+0)/383;c3 = ([120 150 230]+128)/383;patch([0 1 1 0],[0 0 1 1],c1);patch([0 1 1 1-e 1-e 0+e],[0 0 1 1-e 0+e 0+e],c2);patch([0 0 1 1-e 0+e 0+e],[0 1 1 1-e 1-e 0+e],c3);plot([0 1 1 0 0],[0 0 1 1 0]);disp('0');
  "IW{1,1}" : Subsystem
      mask Display: e = 0.06;c1 = [120 150 230]/255;c2 = ([120 150 230]+0)/383;c3 = ([120 150 230]+128)/383;patch([0 1 1 0],[0 0 1 1],c1);patch([0 1 1 1-e 1-e 0+e],[0 0 1 1-e 0+e 0+e],c2);patch([0 0 1 1-e 0+e 0+e],[0 1 1 1-e 1-e 0+e],c3);plot([0 1 1 0 0],[0 0 1 1 0]);disp('W');
  "b{1}" : Constant  Value=[2.00780722196034755455684717162512242794036865234375;-1.614314640024755664882150085759349167346954345703125;1.1634312494625949074844584174570627510547637939453125;0.7159545479146653956803447726997546851634979248046875;0.1978719589126164690728870709790498949587345123291015625;-0.224338082566364171999140353364055044949054718017578125;-0.6089662629231054058465133493882603943347930908203125;-1.143357478345937039421187364496290683746337890625;-1.67809948079147996935489572933875024318695068359375;-2.062226944665316086258144423482008278369903564453125]
      mask Display: e = 0.06;c1 = [120 150 230]/255;c2 = ([120 150 230]+0)/383;c3 = ([120 150 230]+128)/383;patch([0 1 1 0],[0 0 1 1],c1);patch([0 1 1 1-e 1-e 0+e],[0 0 1 1-e 0+e 0+e],c2);patch([0 0 1 1-e 0+e 0+e],[0 1 1 1-e 1-e 0+e],c3);plot([0 1 1 0 0],[0 0 1 1 0]);disp('b');
  netsum : Sum  Inputs=2  InputSameDT=on  SaturateOnIntegerOverflow=on  OutDataTypeStr=Inherit: Same as first input
      mask Display: e = 0.06;c1 = [120 150 230]/255;c2 = ([120 150 230]+0)/383;c3 = ([120 150 230]+128)/383;patch([0 1 1 0],[0 0 1 1],c1);patch([0 1 1 1-e 1-e 0+e],[0 0 1 1-e 0+e 0+e],c2);patch([0 0 1 1-e 0+e 0+e],[0 1 1 1-e 1-e 0+e],c3);plot([0 1 1 0 0],[0 0 1 1 0]);disp('+');
  tansig : neural/Transfer Functions/tansig
  "a{1}" : Outport  InitialOutput=[0;0;0;0;0;0;0;0;0;0]
      mask Display: e = 0.06;c1 = [120 230 180]/255;c2 = ([120 230 180]+0)/(256+128);c3 = ([120 230 180]+128)/(256+128);patch([0 1 1 0],[0 0 1 1],c1);patch([0 1 1 1-e 1-e 0+e],[0 0 1 1-e 0+e 0+e],c2);patch([0 0 1 1-e 0+e 0+e],[0 1 1 1-e 1-e 0+e],c3);plot([0 1 1 0 0],[0 0 1 1 0]);
  wires:
  "p{1}"/1 -> Delays 1/1("p{1}")
  Delays 1/1("pd{1,1}") -> "IW{1,1}"/1("pd{1,1}")
  "IW{1,1}"/1("iz{1,1}") -> netsum/1
  "b{1}"/1 -> netsum/2
  netsum/1 -> tansig/1
  tansig/1 -> "a{1}"/1

== system matlab model/Function Fitting Neural Network1/Layer 2 ==
  "a{1} " : Inport  PortDimensions=10
      mask Display: e = 0.06;c1 = [120 230 180]/255;c2 = ([120 230 180]+0)/(256+128);c3 = ([120 230 180]+128)/(256+128);patch([0 1 1 0],[0 0 1 1],c1);patch([0 1 1 1-e 1-e 0+e],[0 0 1 1-e 0+e 0+e],c2);patch([0 0 1 1-e 0+e 0+e],[0 1 1 1-e 1-e 0+e],c3);plot([0 1 1 0 0],[0 0 1 1 0]);
  Delays 1 : Subsystem
      mask Display: e = 0.06;c1 = [120 150 230]/255;c2 = ([120 150 230]+0)/383;c3 = ([120 150 230]+128)/383;patch([0 1 1 0],[0 0 1 1],c1);patch([0 1 1 1-e 1-e 0+e],[0 0 1 1-e 0+e 0+e],c2);patch([0 0 1 1-e 0+e 0+e],[0 1 1 1-e 1-e 0+e],c3);plot([0 1 1 0 0],[0 0 1 1 0]);disp('0');
  "LW{2,1}" : Subsystem
      mask Display: e = 0.06;c1 = [120 150 230]/255;c2 = ([120 150 230]+0)/383;c3 = ([120 150 230]+128)/383;patch([0 1 1 0],[0 0 1 1],c1);patch([0 1 1 1-e 1-e 0+e],[0 0 1 1-e 0+e 0+e],c2);patch([0 0 1 1-e 0+e 0+e],[0 1 1 1-e 1-e 0+e],c3);plot([0 1 1 0 0],[0 0 1 1 0]);disp('W');
  "b{2}" : Constant  Value=0.0197993567191807016969473664858014672063291072845458984375
      mask Display: e = 0.06;c1 = [120 150 230]/255;c2 = ([120 150 230]+0)/383;c3 = ([120 150 230]+128)/383;patch([0 1 1 0],[0 0 1 1],c1);patch([0 1 1 1-e 1-e 0+e],[0 0 1 1-e 0+e 0+e],c2);patch([0 0 1 1-e 0+e 0+e],[0 1 1 1-e 1-e 0+e],c3);plot([0 1 1 0 0],[0 0 1 1 0]);disp('b');
  netsum : Sum  Inputs=2  InputSameDT=on  SaturateOnIntegerOverflow=on  OutDataTypeStr=Inherit: Same as first input
      mask Display: e = 0.06;c1 = [120 150 230]/255;c2 = ([120 150 230]+0)/383;c3 = ([120 150 230]+128)/383;patch([0 1 1 0],[0 0 1 1],c1);patch([0 1 1 1-e 1-e 0+e],[0 0 1 1-e 0+e 0+e],c2);patch([0 0 1 1-e 0+e 0+e],[0 1 1 1-e 1-e 0+e],c3);plot([0 1 1 0 0],[0 0 1 1 0]);disp('+');
  purelin : neural/Transfer Functions/purelin
  "a{2}" : Outport  InitialOutput=0
      mask Display: e = 0.06;c1 = [120 230 180]/255;c2 = ([120 230 180]+0)/(256+128);c3 = ([120 230 180]+128)/(256+128);patch([0 1 1 0],[0 0 1 1],c1);patch([0 1 1 1-e 1-e 0+e],[0 0 1 1-e 0+e 0+e],c2);patch([0 0 1 1-e 0+e 0+e],[0 1 1 1-e 1-e 0+e],c3);plot([0 1 1 0 0],[0 0 1 1 0]);
  wires:
  "a{1} "/1 -> Delays 1/1("p{2}")
  Delays 1/1("pd{2,1}") -> "LW{2,1}"/1("ad{2,1}")
  "LW{2,1}"/1("lz{2,1}") -> netsum/1
  "b{2}"/1 -> netsum/2
  netsum/1 -> purelin/1
  purelin/1 -> "a{2}"/1

== system matlab model/Function Fitting Neural Network1/Process Input 1 ==
  x : Inport  PortDimensions=6
      mask Display: e = 0.06;c1 = [120 230 180]/255;c2 = ([120 230 180]+0)/(256+128);c3 = ([120 230 180]+128)/(256+128);patch([0 1 1 0],[0 0 1 1],c1);patch([0 1 1 1-e 1-e 0+e],[0 0 1 1-e 0+e 0+e],c2);patch([0 0 1 1-e 0+e 0+e],[0 1 1 1-e 1-e 0+e],c3);plot([0 1 1 0 0],[0 0 1 1 0]);
  mapminmax : neural/Processing Functions/mapminmax  xmin=[0;0;0;0;0;0]  xmax=[1;1;1;1;1;1]  ymin=-1  ymax=1
  p : Outport  PortDimensions=6
      mask Display: e = 0.06;c1 = [120 230 180]/255;c2 = ([120 230 180]+0)/(256+128);c3 = ([120 230 180]+128)/(256+128);patch([0 1 1 0],[0 0 1 1],c1);patch([0 1 1 1-e 1-e 0+e],[0 0 1 1-e 0+e 0+e],c2);patch([0 0 1 1-e 0+e 0+e],[0 1 1 1-e 1-e 0+e],c3);plot([0 1 1 0 0],[0 0 1 1 0]);
  wires:
  x/1 -> mapminmax/1
  mapminmax/1 -> p/1

== system matlab model/Function Fitting Neural Network1/Process Output 1 ==
  a : Inport  PortDimensions=1
      mask Display: e = 0.06;c1 = [120 230 180]/255;c2 = ([120 230 180]+0)/(256+128);c3 = ([120 230 180]+128)/(256+128);patch([0 1 1 0],[0 0 1 1],c1);patch([0 1 1 1-e 1-e 0+e],[0 0 1 1-e 0+e 0+e],c2);patch([0 0 1 1-e 0+e 0+e],[0 1 1 1-e 1-e 0+e],c3);plot([0 1 1 0 0],[0 0 1 1 0]);
  mapminmax_reverse : neural/Processing Functions/mapminmax_reverse  xmin=0  xmax=6  ymin=-1  ymax=1
  y : Outport  PortDimensions=1
      mask Display: e = 0.06;c1 = [120 230 180]/255;c2 = ([120 230 180]+0)/(256+128);c3 = ([120 230 180]+128)/(256+128);patch([0 1 1 0],[0 0 1 1],c1);patch([0 1 1 1-e 1-e 0+e],[0 0 1 1-e 0+e 0+e],c2);patch([0 0 1 1-e 0+e 0+e],[0 1 1 1-e 1-e 0+e],c3);plot([0 1 1 0 0],[0 0 1 1 0]);
  wires:
  a/1 -> mapminmax_reverse/1
  mapminmax_reverse/1 -> y/1

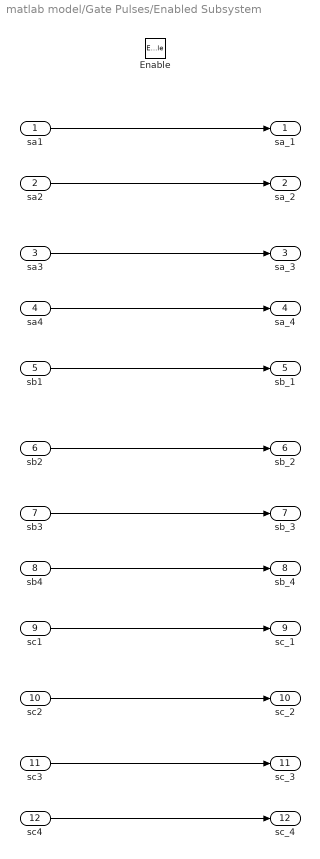
== system matlab model/Gate Pulses/Enabled Subsystem ==
  sa1 : Inport
  sa2 : Inport  Port=2
  sa3 : Inport  Port=3
  sa4 : Inport  Port=4
  sb1 : Inport  Port=5
  sb2 : Inport  Port=6
  sb3 : Inport  Port=7
  sb4 : Inport  Port=8
  sc1 : Inport  Port=9
  sc2 : Inport  Port=10
  sc3 : Inport  Port=11
  sc4 : Inport  Port=12
  Enable : EnablePort
  sa_1 : Outport  VectorParamsAs1DForOutWhenUnconnected=off
  sa_2 : Outport  Port=2  VectorParamsAs1DForOutWhenUnconnected=off
  sa_3 : Outport  Port=3  VectorParamsAs1DForOutWhenUnconnected=off
  sa_4 : Outport  Port=4  VectorParamsAs1DForOutWhenUnconnected=off
  sb_1 : Outport  Port=5  VectorParamsAs1DForOutWhenUnconnected=off
  sb_2 : Outport  Port=6  VectorParamsAs1DForOutWhenUnconnected=off
  sb_3 : Outport  Port=7  VectorParamsAs1DForOutWhenUnconnected=off
  sb_4 : Outport  Port=8  VectorParamsAs1DForOutWhenUnconnected=off
  sc_1 : Outport  Port=9  VectorParamsAs1DForOutWhenUnconnected=off
  sc_2 : Outport  Port=10  VectorParamsAs1DForOutWhenUnconnected=off
  sc_3 : Outport  Port=11  VectorParamsAs1DForOutWhenUnconnected=off
  sc_4 : Outport  Port=12  VectorParamsAs1DForOutWhenUnconnected=off
  wires:
  sa1/1 -> sa_1/1
  sa2/1 -> sa_2/1
  sa3/1 -> sa_3/1
  sa4/1 -> sa_4/1
  sb1/1 -> sb_1/1
  sb2/1 -> sb_2/1
  sb3/1 -> sb_3/1
  sb4/1 -> sb_4/1
  sc1/1 -> sc_1/1
  sc2/1 -> sc_2/1
  sc3/1 -> sc_3/1
  sc4/1 -> sc_4/1

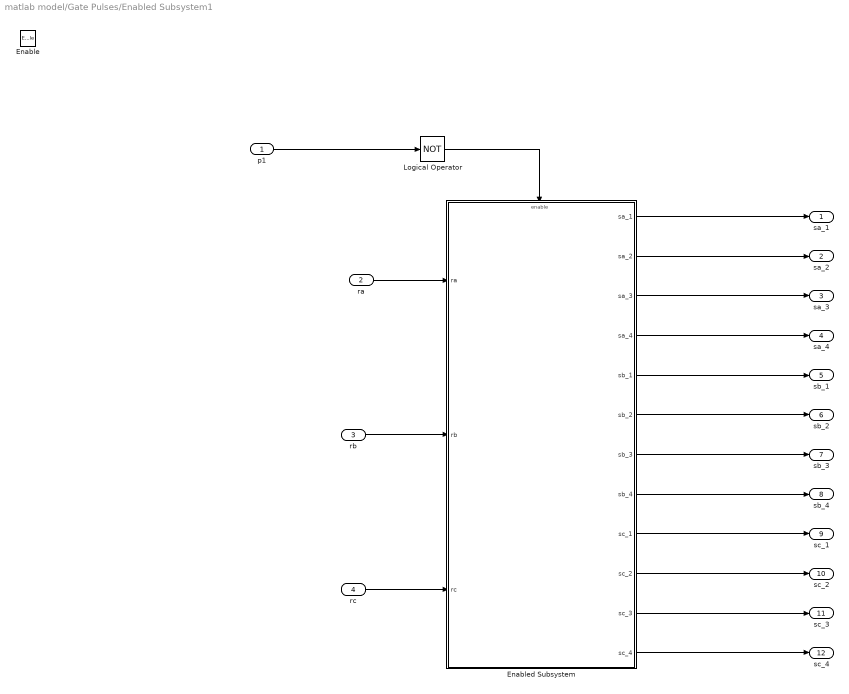
== system matlab model/Gate Pulses/Enabled Subsystem1 ==
  p1 : Inport
  ra : Inport  Port=2
  rb : Inport  Port=3
  rc : Inport  Port=4
  Enable : EnablePort
  Enabled Subsystem : Subsystem  TreatAsAtomicUnit=on
  Logical Operator : Logic  Operator=NOT  AllPortsSameDT=off  OutDataTypeStr=boolean
  sa_1 : Outport  VectorParamsAs1DForOutWhenUnconnected=off
  sa_2 : Outport  Port=2  VectorParamsAs1DForOutWhenUnconnected=off
  sa_3 : Outport  Port=3  VectorParamsAs1DForOutWhenUnconnected=off
  sa_4 : Outport  Port=4  VectorParamsAs1DForOutWhenUnconnected=off
  sb_1 : Outport  Port=5  VectorParamsAs1DForOutWhenUnconnected=off
  sb_2 : Outport  Port=6  VectorParamsAs1DForOutWhenUnconnected=off
  sb_3 : Outport  Port=7  VectorParamsAs1DForOutWhenUnconnected=off
  sb_4 : Outport  Port=8  VectorParamsAs1DForOutWhenUnconnected=off
  sc_1 : Outport  Port=9  VectorParamsAs1DForOutWhenUnconnected=off
  sc_2 : Outport  Port=10  VectorParamsAs1DForOutWhenUnconnected=off
  sc_3 : Outport  Port=11  VectorParamsAs1DForOutWhenUnconnected=off
  sc_4 : Outport  Port=12  VectorParamsAs1DForOutWhenUnconnected=off
  wires:
  p1/1 -> Logical Operator/1
  Logical Operator/1 -> Enabled Subsystem/Enable
  ra/1 -> Enabled Subsystem/1(ra)
  rb/1 -> Enabled Subsystem/2(rb)
  rc/1 -> Enabled Subsystem/3(rc)
  Enabled Subsystem/1(sa_1) -> sa_1/1
  Enabled Subsystem/2(sa_2) -> sa_2/1
  Enabled Subsystem/3(sa_3) -> sa_3/1
  Enabled Subsystem/4(sa_4) -> sa_4/1
  Enabled Subsystem/5(sb_1) -> sb_1/1
  Enabled Subsystem/6(sb_2) -> sb_2/1
  Enabled Subsystem/7(sb_3) -> sb_3/1
  Enabled Subsystem/8(sb_4) -> sb_4/1
  Enabled Subsystem/9(sc_1) -> sc_1/1
  Enabled Subsystem/10(sc_2) -> sc_2/1
  Enabled Subsystem/11(sc_3) -> sc_3/1
  Enabled Subsystem/12(sc_4) -> sc_4/1

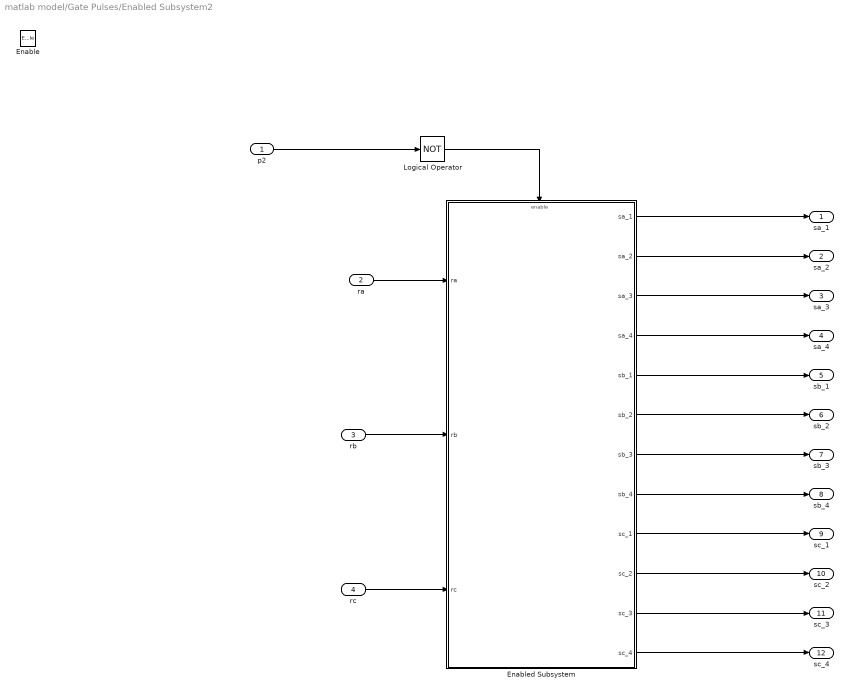
== system matlab model/Gate Pulses/Enabled Subsystem2 ==
  p2 : Inport
  ra : Inport  Port=2
  rb : Inport  Port=3
  rc : Inport  Port=4
  Enable : EnablePort
  Enabled Subsystem : Subsystem  TreatAsAtomicUnit=on
  Logical Operator : Logic  Operator=NOT  AllPortsSameDT=off  OutDataTypeStr=boolean
  sa_1 : Outport  VectorParamsAs1DForOutWhenUnconnected=off
  sa_2 : Outport  Port=2  VectorParamsAs1DForOutWhenUnconnected=off
  sa_3 : Outport  Port=3  VectorParamsAs1DForOutWhenUnconnected=off
  sa_4 : Outport  Port=4  VectorParamsAs1DForOutWhenUnconnected=off
  sb_1 : Outport  Port=5  VectorParamsAs1DForOutWhenUnconnected=off
  sb_2 : Outport  Port=6  VectorParamsAs1DForOutWhenUnconnected=off
  sb_3 : Outport  Port=7  VectorParamsAs1DForOutWhenUnconnected=off
  sb_4 : Outport  Port=8  VectorParamsAs1DForOutWhenUnconnected=off
  sc_1 : Outport  Port=9  VectorParamsAs1DForOutWhenUnconnected=off
  sc_2 : Outport  Port=10  VectorParamsAs1DForOutWhenUnconnected=off
  sc_3 : Outport  Port=11  VectorParamsAs1DForOutWhenUnconnected=off
  sc_4 : Outport  Port=12  VectorParamsAs1DForOutWhenUnconnected=off
  wires:
  Enabled Subsystem/12(sc_4) -> sc_4/1
  Enabled Subsystem/11(sc_3) -> sc_3/1
  Enabled Subsystem/10(sc_2) -> sc_2/1
  Enabled Subsystem/9(sc_1) -> sc_1/1
  Enabled Subsystem/8(sb_4) -> sb_4/1
  Enabled Subsystem/7(sb_3) -> sb_3/1
  Enabled Subsystem/6(sb_2) -> sb_2/1
  Enabled Subsystem/5(sb_1) -> sb_1/1
  Enabled Subsystem/4(sa_4) -> sa_4/1
  Enabled Subsystem/3(sa_3) -> sa_3/1
  Enabled Subsystem/2(sa_2) -> sa_2/1
  Enabled Subsystem/1(sa_1) -> sa_1/1
  rc/1 -> Enabled Subsystem/3(rc)
  rb/1 -> Enabled Subsystem/2(rb)
  ra/1 -> Enabled Subsystem/1(ra)
  Logical Operator/1 -> Enabled Subsystem/Enable
  p2/1 -> Logical Operator/1

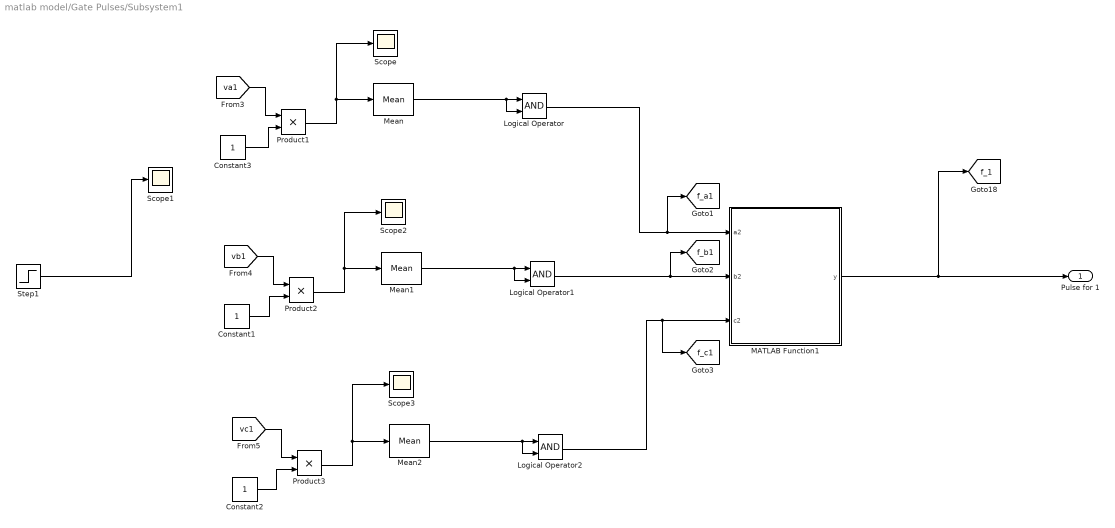
== system matlab model/Gate Pulses/Subsystem1 ==
  Constant1 : Constant
  Constant2 : Constant
  Constant3 : Constant
  Logical Operator : Logic  AllPortsSameDT=off  OutDataTypeStr=boolean
  Logical Operator1 : Logic  AllPortsSameDT=off  OutDataTypeStr=boolean
  Logical Operator2 : Logic  AllPortsSameDT=off  OutDataTypeStr=boolean
  MATLAB Function1 : MATLAB Function  TreatAsAtomicUnit=on
  Mean : spsMeanLib/Mean  Freq=50  Vinit=1  Ts=0
  Mean1 : spsMeanLib/Mean  Freq=50  Vinit=1  Ts=0
  Mean2 : spsMeanLib/Mean  Freq=50  Vinit=1  Ts=0
  Product1 : Product
  Product2 : Product
  Product3 : Product
  Scope{,1..3} (4 alike) : Scope
  Step1 : Step  Time=0.04  Before=1  After=0  SampleTime=0
  Pulse for 1 : Outport  VectorParamsAs1DForOutWhenUnconnected=off
  tag scope: f_1=global, f_a1=global, f_b1=global, f_c1=global
  wires:
  Logical Operator/1 -> MATLAB Function1/1(a2), [f_a1]
  Mean/1 -> Logical Operator/1, Logical Operator/2
  Product1/1 -> Scope/1, Mean/1
  Mean1/1 -> Logical Operator1/2, Logical Operator1/1
  [vb1] -> Product2/1
  Logical Operator1/1 -> [f_b1], MATLAB Function1/2(b2)
  Product2/1 -> Mean1/1, Scope2/1
  Mean2/1 -> Logical Operator2/1, Logical Operator2/2
  [vc1] -> Product3/1
  Product3/1 -> Scope3/1, Mean2/1
  Logical Operator2/1 -> [f_c1], MATLAB Function1/3(c2)
  MATLAB Function1/1(y) -> [f_1], Pulse for 1/1
  [va1] -> Product1/1
  Step1/1 -> Scope1/1
  Constant3/1 -> Product1/2
  Constant2/1 -> Product3/2
  Constant1/1 -> Product2/2

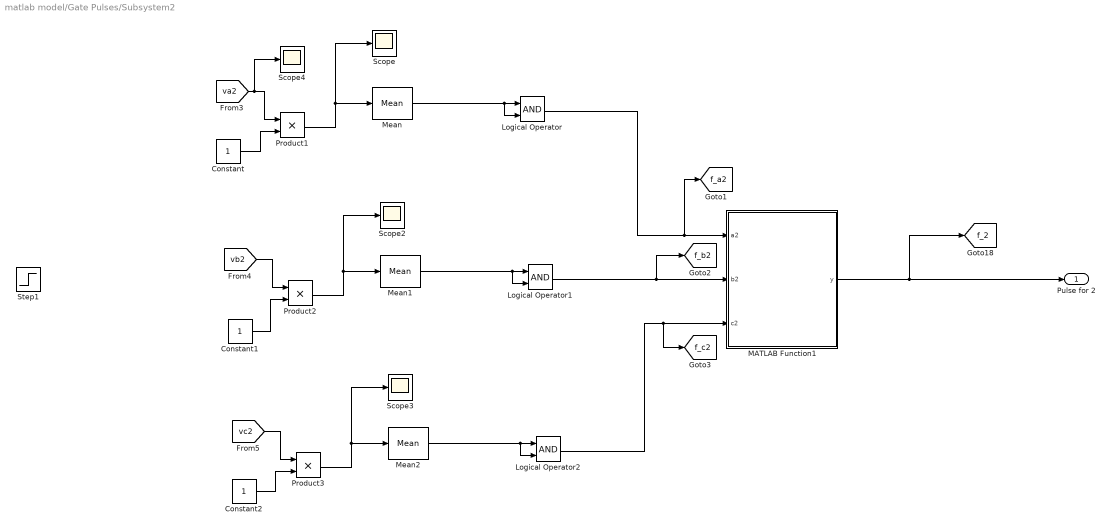
== system matlab model/Gate Pulses/Subsystem2 ==
  Constant : Constant
  Constant1 : Constant
  Constant2 : Constant
  Logical Operator : Logic  AllPortsSameDT=off  OutDataTypeStr=boolean
  Logical Operator1 : Logic  AllPortsSameDT=off  OutDataTypeStr=boolean
  Logical Operator2 : Logic  AllPortsSameDT=off  OutDataTypeStr=boolean
  MATLAB Function1 : MATLAB Function  TreatAsAtomicUnit=on
  Mean : spsMeanLib/Mean  Freq=50  Vinit=1  Ts=0
  Mean1 : spsMeanLib/Mean  Freq=50  Vinit=1  Ts=0
  Mean2 : spsMeanLib/Mean  Freq=50  Vinit=1  Ts=0
  Product1 : Product
  Product2 : Product
  Product3 : Product
  Scope{,2..4} (4 alike) : Scope
  Step1 : Step  Time=0.04  Before=1  After=0  SampleTime=0
  Pulse for 2 : Outport  VectorParamsAs1DForOutWhenUnconnected=off
  tag scope: f_2=global, f_a2=global, f_b2=global, f_c2=global
  wires:
  [va2] -> Scope4/1, Product1/1
  Constant/1 -> Product1/2
  Constant2/1 -> Product3/2
  Logical Operator2/1 -> [f_c2], MATLAB Function1/3(c2)
  Product3/1 -> Mean2/1, Scope3/1
  [vc2] -> Product3/1
  Mean2/1 -> Logical Operator2/2, Logical Operator2/1
  Product2/1 -> Scope2/1, Mean1/1
  Logical Operator1/1 -> [f_b2], MATLAB Function1/2(b2)
  [vb2] -> Product2/1
  Mean1/1 -> Logical Operator1/1, Logical Operator1/2
  Product1/1 -> Mean/1, Scope/1
  Mean/1 -> Logical Operator/2, Logical Operator/1
  Logical Operator/1 -> [f_a2], MATLAB Function1/1(a2)
  MATLAB Function1/1(y) -> [f_2], Pulse for 2/1
  Constant1/1 -> Product2/2

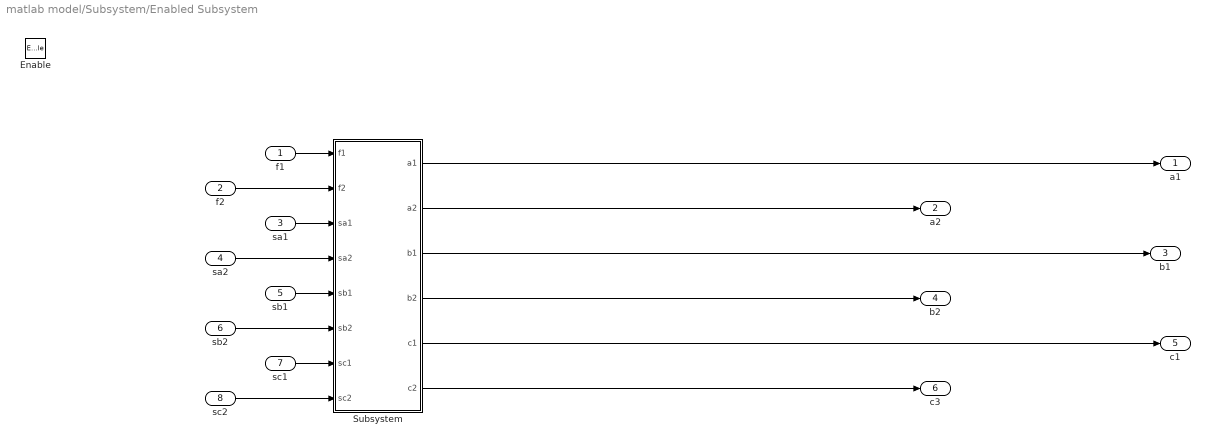
== system matlab model/Subsystem/Enabled Subsystem ==
  f1 : Inport
  f2 : Inport  Port=2
  sa1 : Inport  Port=3
  sa2 : Inport  Port=4
  sb1 : Inport  Port=5
  sb2 : Inport  Port=6
  sc1 : Inport  Port=7
  sc2 : Inport  Port=8
  Enable : EnablePort
  Subsystem : Subsystem
  a1 : Outport  VectorParamsAs1DForOutWhenUnconnected=off
  a2 : Outport  Port=2  VectorParamsAs1DForOutWhenUnconnected=off
  b1 : Outport  Port=3  VectorParamsAs1DForOutWhenUnconnected=off
  b2 : Outport  Port=4  VectorParamsAs1DForOutWhenUnconnected=off
  c1 : Outport  Port=5  VectorParamsAs1DForOutWhenUnconnected=off
  c3 : Outport  Port=6  VectorParamsAs1DForOutWhenUnconnected=off
  wires:
  Subsystem/1(a1) -> a1/1
  Subsystem/6(c2) -> c3/1
  Subsystem/5(c1) -> c1/1
  Subsystem/4(b2) -> b2/1
  Subsystem/3(b1) -> b1/1
  Subsystem/2(a2) -> a2/1
  f1/1 -> Subsystem/1(f1)
  f2/1 -> Subsystem/2(f2)
  sa1/1 -> Subsystem/3(sa1)
  sa2/1 -> Subsystem/4(sa2)
  sb1/1 -> Subsystem/5(sb1)
  sb2/1 -> Subsystem/6(sb2)
  sc1/1 -> Subsystem/7(sc1)
  sc2/1 -> Subsystem/8(sc2)

== system matlab model/Function Fitting Neural Network1/Layer 1/Delays 1 ==
  "p{1}" : Inport  PortDimensions=6
      mask Display: e = 0.06;c1 = [120 230 180]/255;c2 = ([120 230 180]+0)/(256+128);c3 = ([120 230 180]+128)/(256+128);patch([0 1 1 0],[0 0 1 1],c1);patch([0 1 1 1-e 1-e 0+e],[0 0 1 1-e 0+e 0+e],c2);patch([0 0 1 1-e 0+e 0+e],[0 1 1 1-e 1-e 0+e],c3);plot([0 1 1 0 0],[0 0 1 1 0]);
  mux : Mux  Inputs=1
      mask Display: e = 0.06;c1 = [120 150 230]/255;c2 = ([120 150 230]+0)/383;c3 = ([120 150 230]+128)/383;patch([0 1 1 0],[0 0 1 1],c1);patch([0 1 1 1-e 1-e 0+e],[0 0 1 1-e 0+e 0+e],c2);patch([0 0 1 1-e 0+e 0+e],[0 1 1 1-e 1-e 0+e],c3);plot([0 1 1 0 0],[0 0 1 1 0]);disp('Mux')
  "pd{1,1}" : Outport
      mask Display: e = 0.06;c1 = [120 230 180]/255;c2 = ([120 230 180]+0)/(256+128);c3 = ([120 230 180]+128)/(256+128);patch([0 1 1 0],[0 0 1 1],c1);patch([0 1 1 1-e 1-e 0+e],[0 0 1 1-e 0+e 0+e],c2);patch([0 0 1 1-e 0+e 0+e],[0 1 1 1-e 1-e 0+e],c3);plot([0 1 1 0 0],[0 0 1 1 0]);
  wires:
  "p{1}"/1 -> mux/1
  mux/1 -> "pd{1,1}"/1
